simulink model "Part2_A"  (R2025b)
settings: Solver=VariableStepAuto  StartTime=0.0  StopTime=20  RelTol=1e-3
settings Model: Creator=hahnc  LastModifiedBy=hahnc

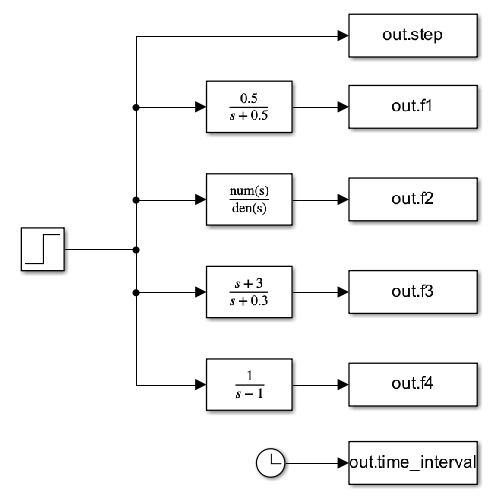
[thumbnail: Simulink's stored preview of the top-level diagram]
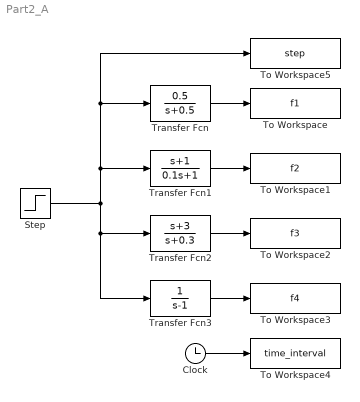
== system Part2_A ==
  Clock : Clock
  Step : Step  SampleTime=0
  To Workspace : ToWorkspace  VariableName=f1  SampleTime=-1
  To Workspace1 : ToWorkspace  VariableName=f2  SampleTime=-1
  To Workspace2 : ToWorkspace  VariableName=f3  SampleTime=-1
  To Workspace3 : ToWorkspace  VariableName=f4  SampleTime=-1
  To Workspace4 : ToWorkspace  VariableName=time_interval  SampleTime=-1
  To Workspace5 : ToWorkspace  VariableName=step  SampleTime=-1
  Transfer Fcn : TransferFcn  Numerator=[0.5]  Denominator=[1 0.5]
  Transfer Fcn1 : TransferFcn  Numerator=[1 1]  Denominator=[0.1 1]
  Transfer Fcn2 : TransferFcn  Numerator=[1 3]  Denominator=[1 0.3]
  Transfer Fcn3 : TransferFcn  Denominator=[1 -1]
  wires:
  Step/1 -> Transfer Fcn3/1, Transfer Fcn2/1, Transfer Fcn1/1, To Workspace5/1, Transfer Fcn/1
  Transfer Fcn/1 -> To Workspace/1
  Transfer Fcn1/1 -> To Workspace1/1
  Transfer Fcn2/1 -> To Workspace2/1
  Transfer Fcn3/1 -> To Workspace3/1
  Clock/1 -> To Workspace4/1
